simulink model "RLC2"  (R2024b)
settings: Solver=VariableStepAuto  StartTime=0.0  StopTime=100.0  FixedStep=0.0001  RelTol=1e-3
settings Model: Creator=castl  LastModifiedBy=castl

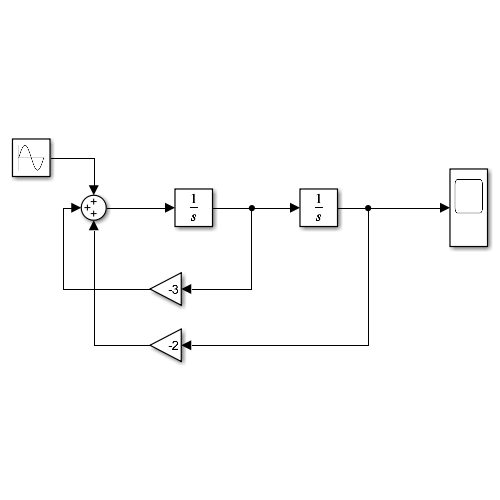
[thumbnail: Simulink's stored preview of the top-level diagram]
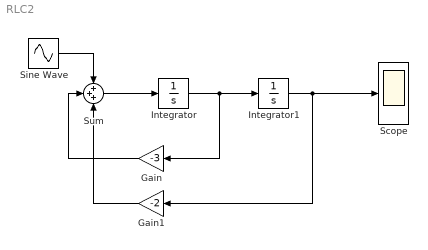
== system RLC2 ==
  Gain : Gain  Gain=-3
  Gain1 : Gain  Gain=-2
  Integrator : Integrator
  Integrator1 : Integrator
  Scope : Scope
  Sine Wave : Sin  Amplitude=5  Phase=pi/4  SampleTime=0
  Sum : Sum  Inputs=+++
  wires:
  Sine Wave/1 -> Sum/1
  Sum/1 -> Integrator/1
  Integrator/1 -> Gain/1, Integrator1/1
  Integrator1/1 -> Gain1/1, Scope/1
  Gain/1 -> Sum/2
  Gain1/1 -> Sum/3
